simulink model "Suspension_PID"  (R2023b)
settings: Solver=VariableStepAuto  StartTime=0.0  StopTime=10.0  RelTol=1e-3
values from neighbouring files (symbols this model uses):
  b1 = 350    [Suspension_Model_PID.m]
  b2 = 15020    [Suspension_Model_PID.m]
  k1 = 80000    [Suspension_Model_PID.m]
  k2 = 500000    [Suspension_Model_PID.m]
  Kd = 210000    [Suspension_Model_PID.m]
  Ki = 1200000    [Suspension_Model_PID.m]
  Kp = 835000    [Suspension_Model_PID.m]
  m1 = 2500    [Suspension_Model_PID.m]
  m2 = 320    [Suspension_Model_PID.m]
libraries: slpidlib x1
settings Model: Creator=mdhel  LastModifiedBy=mdhel

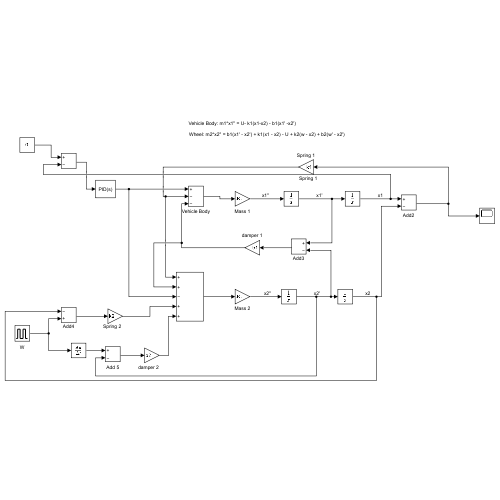
[thumbnail: Simulink's stored preview of the top-level diagram]
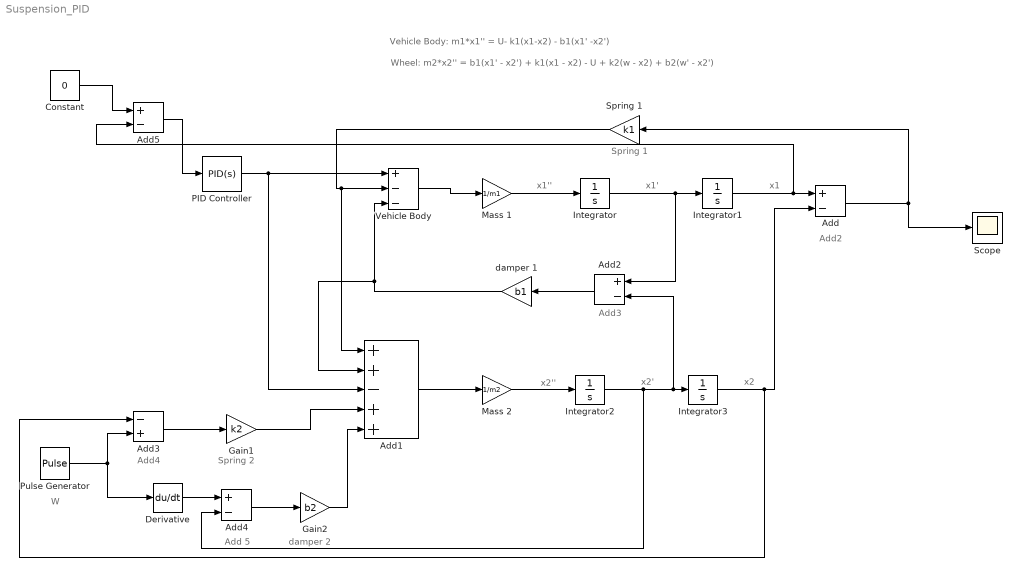
== system Suspension_PID ==
  note: Wheel: m2*x2'' = b1(x1' - x2') + k1(x1 - x2) - U + k2(w - x2) + b2(w' - x2')
  note: Vehicle Body: m1*x1'' = U- k1(x1-x2) - b1(x1' -x2')
  note: x1'
  note: x2'
  note: x2
  note: W
  note: Add4
  note: damper 2
  note: Spring 1
  note: Add2
  note: Add 5
  note: x2''
  note: Add3
  note: x1
  note: x1''
  note: Spring 2
  Add{,2,4..5} (4 alike) : Sum  Inputs=+-
  Add1 : Sum  Inputs=++-++
  Add3 : Sum  Inputs=-+
  Constant : Constant  Value=0
  Derivative : Derivative
  Gain1 : Gain  Gain=k2
  Gain2 : Gain  Gain=b2
  Integrator{,1..3} (4 alike) : Integrator
  Mass 1 : Gain  Gain=1/m1
  Mass 2 : Gain  Gain=1/m2
  PID Controller : slpidlib/PID Controller  Controller=PID  Form=Parallel  TimeDomain=Continuous-time  UseExternalTs=off  SampleTime=-1  IntegratorMethod=Forward Euler  FilterMethod=Forward Euler  ControllerParametersSource=internal  P=Kp  I=Ki  UseKiTs=off  D=Kd  N=100  UseFilter=on  TunerSelectOption=Transfer Function Based (PID Tuner App)  InitialConditionSource=internal  InitialConditionForIntegrator=0  InitialConditionForFilter=0  DifferentiatorICPrevScaledInput=0  ExternalReset=none  TrackingMode=off  Kt=1  LimitOutput=off  SatLimitsSource=internal  UpperSaturationLimit=inf  LowerSaturationLimit=-inf  LinearizeAsGain=on  AntiWindupMode=none  Kb=1  LimitIntegrator=off  UpperIntegratorSaturationLimit=inf  LowerIntegratorSaturationLimit=-inf  POutMin=[]  POutMax=[]  IOutMin=[]  IOutMax=[]  DOutMin=[]  DOutMax=[]  NOutMin=[]  NOutMax=[]  SumOutMin=[]  SumOutMax=[]  SaturationOutMin=[]  SaturationOutMax=[]  PParamMin=[]  PParamMax=[]  IParamMin=[]  IParamMax=[]  DParamMin=[]  DParamMax=[]  NParamMin=[]  NParamMax=[]  KbParamMin=[]  KbParamMax=[]  KtParamMin=[]  KtParamMax=[]  KbOutMin=[]  KbOutMax=[]  KtOutMin=[]  KtOutMax=[]  IntegratorOutMin=[]  IntegratorOutMax=[]  FilterOutMin=[]  FilterOutMax=[]  SumI1OutMin=[]  SumI1OutMax=[]  SumI2OutMin=[]  SumI2OutMax=[]  SumI3OutMin=[]  SumI3OutMax=[]  SumI4OutMin=[]  SumI4OutMax=[]  SumDOutMin=[]  SumDOutMax=[]  DifferentiatorOutMin=[]  DifferentiatorOutMax=[]  FilterDiffOutCoefMin=[]  FilterDiffOutCoefMax=[]  ReciprocalOutMin=[]  ReciprocalOutMax=[]  SumDenOutMin=[]  SumDenOutMax=[]  SumNumOutMin=[]  SumNumOutMax=[]  DivideOutMin=[]  DivideOutMax=[]  UdiffTsProdOutMin=[]  UdiffTsProdOutMax=[]  NTsProdOutMin=[]  NTsProdOutMax=[]  UintegralTsProdOutMin=[]  UintegralTsProdOutMax=[]  UngainTsProdOutMin=[]  UngainTsProdOutMax=[]  ClampingZeroOutDataTypeStr=Inherit: Inherit via back propagation  ClampingZeroOutMin=[]  ClampingZeroOutMax=[]  FilterDenConstantOutDataTypeStr=Inherit: Inherit via back propagation  FilterDenConstantOutMin=[]  FilterDenConstantOutMax=[]  PCopyOutDataTypeStr=Inherit: Inherit via back propagation  PCopyOutMin=[]  PCopyOutMax=[]  NCopyOutDataTypeStr=Inherit: Inherit via back propagation  NCopyOutMin=[]  NCopyOutMax=[]  IntegratorContinuousStateAttributes=''  IntegratorStateMustResolveToSignalObject=off  IntegratorRTWStateStorageClass=Auto  FilterContinuousStateAttributes=''  FilterStateMustResolveToSignalObject=off  FilterRTWStateStorageClass=Auto  ParallelPVariant=InternalParameters  IdealPVariant=Disabled  IVariant=InternalParameters  DVariant=InternalParameters  IntegratorVariant=Continuous  SatVariant=Disabled  AWVariant=Passthrough  PCopyVariant=Disabled  TRVariant=Disabled  FdbkBlocksVariant=Forward  IdealPFdbkVariant=Disabled  SatFdbkVariant=Disabled  DerivativeFilterVariant=ContFilter  NVariant=InternalParameters  NCopyVariant=Disabled  FilterICVariant=InternalICsFilter  IntegratorICVariant=InternalICs  ExternalResetVariant=Disabled  TRSumVariant=Passthrough  SumFdbkVariant=Disabled  SumVariant=Sum_PID  TsampFilterVariant=InternalTs  TsampNgainVariant=Passthrough  TsampIntegralVariant=Disabled_SignalSpec  ExternalSaturationOutDataTypeStr=Inherit: Same as second input
  Pulse Generator : DiscretePulseGenerator  PulseType=Time based  Amplitude=0.1  Period=10  PulseWidth=10  PhaseDelay=1
  Scope : Scope
  Spring 1 : Gain  Gain=k1
  Vehicle Body : Sum  Inputs=+--
  damper 1 : Gain  Gain=b1
  wires:
  Integrator3/1 -> Add3/1, Add/2
  Integrator/1 -> Add2/1, Integrator1/1
  Vehicle Body/1 -> Mass 1/1
  PID Controller/1 -> Add1/3, Vehicle Body/1
  Mass 2/1 -> Integrator2/1
  Add/1 -> Spring 1/1, Scope/1
  Gain2/1 -> Add1/5
  damper 1/1 -> Add1/2, Vehicle Body/3
  Mass 1/1 -> Integrator/1
  Derivative/1 -> Add4/1
  Pulse Generator/1 -> Add3/2, Derivative/1
  Add4/1 -> Gain2/1
  Integrator1/1 -> Add5/2, Add/1
  Gain1/1 -> Add1/4
  Add3/1 -> Gain1/1
  Add2/1 -> damper 1/1
  Integrator2/1 -> Add4/2, Add2/2, Integrator3/1
  Add1/1 -> Mass 2/1
  Spring 1/1 -> Add1/1, Vehicle Body/2
  Constant/1 -> Add5/1
  Add5/1 -> PID Controller/1
